simulink library "btnb"  (Simulink 8.1)
settings: Solver=ode1  StartTime=0.0  StopTime=Inf  FixedStep=0.001  RelTol=1e-3
PostLoadFcn:
  | , if any(exist('dsrtsu_mdlpostloadfcn', 'file') == [2, 3, 6]), try dsrtsu_mdlpostloadfcn('Execute', bdroot); catch fprintf('Error in PostLoadFcn (dsrtsu_mdlpostloadfcn) for model "%s":\n %s\n', bdroot, lasterr); end, end,
undefined symbols (not defined in the file or in its folder): KACC_ACCDefBrakDist_m, KACC_BrakeToStopFreeRunTime_s, KACC_SlowTargetConsideredDecel_mps2
libraries: hcu_lib x1
settings Model: DSRTSU_INTERNAL_RTI_VER=450  DSRTSU_INTERNAL_RTI_TYPE=rti1401  Creator=AT015555  LastModifiedBy=AT015555

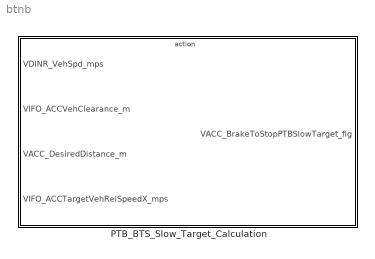
== system btnb ==
  PTB_BTS_Slow_Target_Calculation : Subsystem  TreatAsAtomicUnit=on

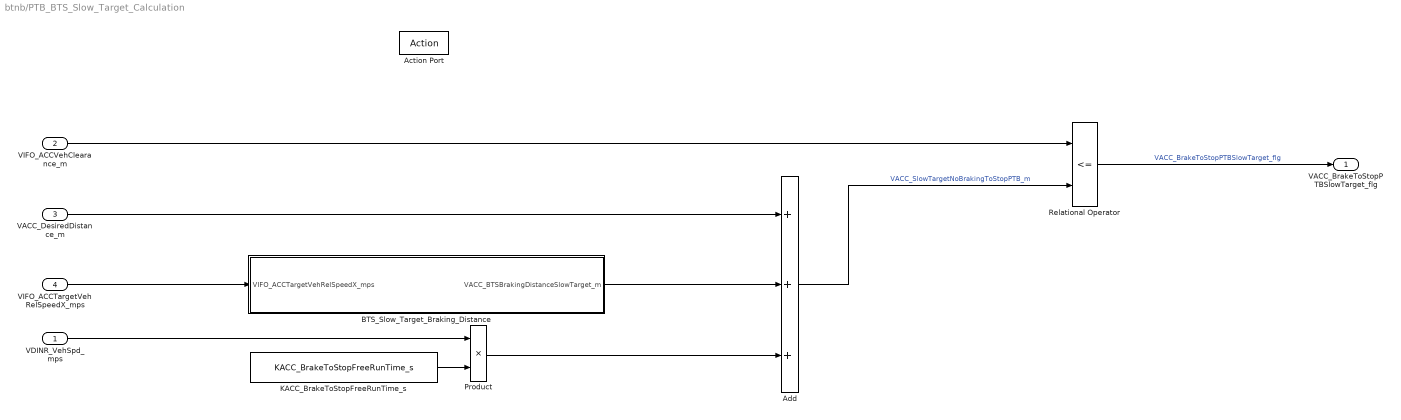
== system btnb/PTB_BTS_Slow_Target_Calculation ==
  VDINR_VehSpd_mps : Inport
  VIFO_ACCVehClearance_m : Inport  Port=2
  VACC_DesiredDistance_m : Inport  Port=3
  VIFO_ACCTargetVehRelSpeedX_mps : Inport  Port=4
  Action Port : ActionPort
  Add : Sum  Inputs=+++
  BTS_Slow_Target_Braking_Distance : Subsystem
  KACC_BrakeToStopFreeRunTime_s : Constant  Value=KACC_BrakeToStopFreeRunTime_s
  Product : Product
  Relational Operator : RelationalOperator  Operator=<=  OutDataTypeStr=boolean
  VACC_BrakeToStopPTBSlowTarget_flg : Outport
  wires:
  VIFO_ACCVehClearance_m/1 -> Relational Operator/1
  VDINR_VehSpd_mps/1 -> Product/1
  BTS_Slow_Target_Braking_Distance/1(VACC_BTSBrakingDistanceSlowTarget_m) -> Add/2
  KACC_BrakeToStopFreeRunTime_s/1 -> Product/2
  Product/1 -> Add/3
  Add/1 -> Relational Operator/2  "VACC_SlowTargetNoBrakingToStopPTB_m"
  Relational Operator/1 -> VACC_BrakeToStopPTBSlowTarget_flg/1  "VACC_BrakeToStopPTBSlowTarget_flg"
  VIFO_ACCTargetVehRelSpeedX_mps/1 -> BTS_Slow_Target_Braking_Distance/1(VIFO_ACCTargetVehRelSpeedX_mps)
  VACC_DesiredDistance_m/1 -> Add/1

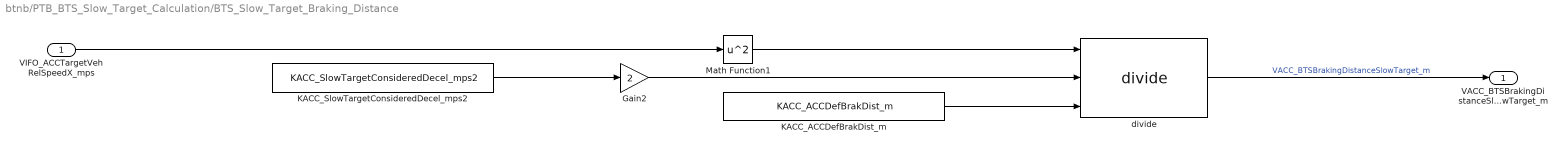
== system btnb/PTB_BTS_Slow_Target_Calculation/BTS_Slow_Target_Braking_Distance ==
  VIFO_ACCTargetVehRelSpeedX_mps : Inport
  Gain2 : Gain  Gain=2
  KACC_ACCDefBrakDist_m : Constant  Value=KACC_ACCDefBrakDist_m
  KACC_SlowTargetConsideredDecel_mps2 : Constant  Value=KACC_SlowTargetConsideredDecel_mps2
  Math Function1 : Math  Operator=square  SaturateOnIntegerOverflow=on
  divide : hcu_lib/divide
  VACC_BTSBrakingDistanceSlowTarget_m : Outport
  wires:
  Math Function1/1 -> divide/1
  Gain2/1 -> divide/2
  KACC_ACCDefBrakDist_m/1 -> divide/3
  VIFO_ACCTargetVehRelSpeedX_mps/1 -> Math Function1/1
  divide/1 -> VACC_BTSBrakingDistanceSlowTarget_m/1  "VACC_BTSBrakingDistanceSlowTarget_m"
  KACC_SlowTargetConsideredDecel_mps2/1 -> Gain2/1
